simulink model "Simulink_one_rotor"  (R2024b)
settings: Solver=VariableStepAuto  StartTime=0.0  StopTime=0.5  RelTol=1e-3
settings Model: Creator=yuany  LastModifiedBy=yuany

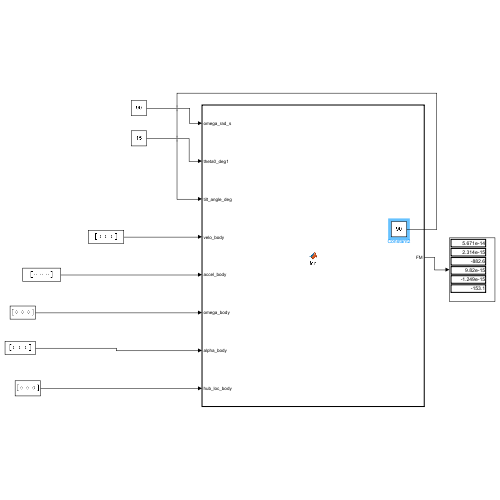
[thumbnail: Simulink's stored preview of the top-level diagram]
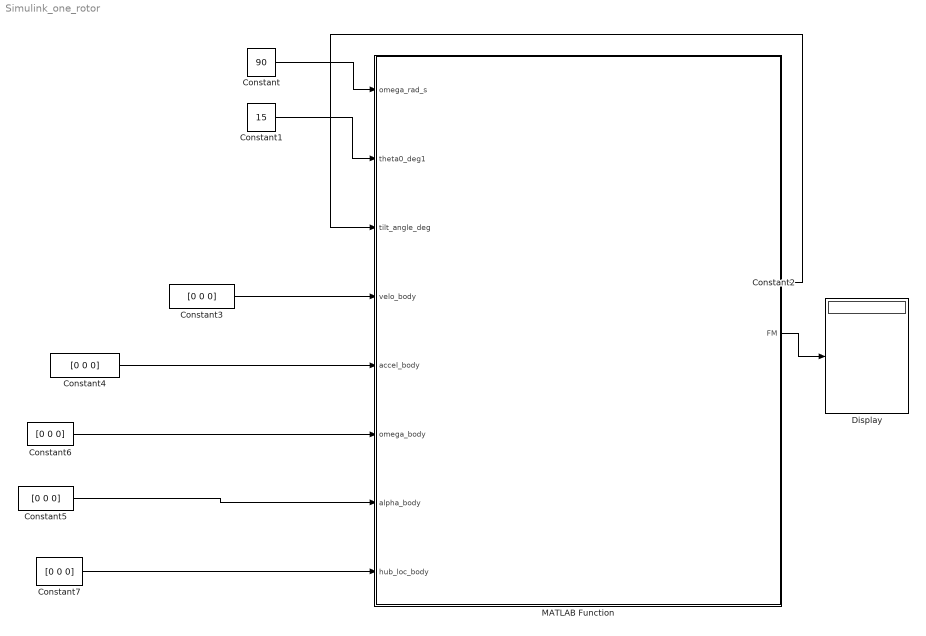
== system Simulink_one_rotor ==
  Constant : Constant  Value=90
  Constant1 : Constant  Value=15
  Constant2 : Constant  Value=90
  Constant{3..7} (5 alike) : Constant  Value=[0 0 0]
  Display : Display
  MATLAB Function : MATLAB Function  TreatAsAtomicUnit=on
  wires:
  Constant/1 -> MATLAB Function/1(omega_rad_s)
  Constant1/1 -> MATLAB Function/2(theta0_deg1)
  Constant2/1 -> MATLAB Function/3(tilt_angle_deg)
  Constant3/1 -> MATLAB Function/4(velo_body)
  Constant4/1 -> MATLAB Function/5(accel_body)
  Constant5/1 -> MATLAB Function/7(alpha_body)
  Constant6/1 -> MATLAB Function/6(omega_body)
  MATLAB Function/1(FM) -> Display/1
  Constant7/1 -> MATLAB Function/8(hub_loc_body)

== matlab function Simulink_one_rotor/MATLAB Function ==
  data: omega_rad_s input; FM output; theta0_deg1 input; tilt_angle_deg input; velo_body input; accel_body input; omega_body input; alpha_body input; hub_loc_body input
function FM = fcn(omega_rad_s, theta0_deg1, tilt_angle_deg, ... 
    velo_body, accel_body, omega_body, alpha_body, hub_loc_body) 
ff=load('rotor.mat');
rotor=ff.rotor;
velo_body = velo_body';
angular_velocity_body = omega_body';
acceleration_body = accel_body';
angular_acceleration_body = alpha_body';
rotor.omega=omega_rad_s;
rotor.tilt_angle_deg=tilt_angle_deg;
rotor.hub_loc=hub_loc_body';

%% Rotor definition
max_id = 6;

%% Control input
theta0_deg = theta0_deg1;

%% Solver options
max_iter = 40;
tol = 1e-10;
fd_step = 1e-4;
damping = 1.0;
min_damping = 0.15;
initial_guess = [zeros(2*rotor.Nb,1); 1.0];

%% Solve
[forces, converged, iter, residual, residual_norm, power, vi, ...
    beta0, dbeta0, beta_hist, dbeta_hist, alpha_hist] = ...
    rotor_bemt_trim_flat_codegen_ready( ...
        rotor, ...
        velo_body, angular_velocity_body, acceleration_body, angular_acceleration_body, ...
        theta0_deg, ...
        max_iter, tol, fd_step, damping, min_damping, initial_guess);

FM=forces;
end

function [forces, converged, iter, residual, residual_norm, power, vi, beta0, dbeta0, beta_hist, dbeta_hist, alpha_hist] = ...
    rotor_bemt_trim_flat_codegen_ready( ...
        rotor, ...
        velo_body, angular_velocity_body, acceleration_body, angular_acceleration_body, ...
        theta0_deg, ...
        max_iter, tol, fd_step, damping, min_damping, initial_guess)
% rotor_bemt_trim_flat_codegen_ready
%
% Code-generation-friendly BEMT + flap trim core.
%
% Runtime restrictions intentionally enforced:
%   - only one struct is used: rotor
%   - no state/options/info/aux/flow_state structs
%   - no try/catch
%   - no function_handle
%   - no griddedInterpolant
%   - no runtime file I/O
%   - no runtime text parsing / MAT loading
%
% Model selection is numeric:
%   rotor.airfoil_mode_code  : 1 linear, 2 lookup table
%   rotor.chord_mode_code    : 1 linear, 2 lookup table
%   rotor.chord_unit_code    : 1 meter, 2 c_over_R
%   rotor.pretwist_mode_code : 1 linear, 2 lookup table
%
% For lookup mode, the corresponding numeric arrays must already be stored
% in rotor before calling this function.

    x = initial_guess(:);
    converged = false;

    for iter = 1:max_iter
        [residual, forces, power, beta_hist, dbeta_hist, alpha_hist, ...
            Tb_average, V_inf, V_infy, V_z] = ...
            rotor_trim_residual_flat_codegen( ...
                x, rotor, ...
                velo_body, angular_velocity_body, acceleration_body, angular_acceleration_body, ...
                theta0_deg);

        resnorm = norm(residual);

        if resnorm < tol
            converged = true;
            break;
        end

        n = numel(x);
        J = zeros(n, n);
        for i = 1:n
            dx = fd_step * max(1.0, abs(x(i)));
            xp = x;
            xp(i) = xp(i) + dx;

            rp = rotor_trim_residual_flat_codegen( ...
                xp, rotor, ...
                velo_body, angular_velocity_body, acceleration_body, angular_acceleration_body, ...
                theta0_deg);

            J(:, i) = (rp - residual) / dx;
        end

        step = -J \ residual;

        alpha = damping;
        accepted = false;
        for ls = 1:8
            x_try = x + alpha * step;

            r_try = rotor_trim_residual_flat_codegen( ...
                x_try, rotor, ...
                velo_body, angular_velocity_body, acceleration_body, angular_acceleration_body, ...
                theta0_deg);

            if norm(r_try) < resnorm
                x = x_try;
                accepted = true;
                break;
            end

            alpha = alpha * 0.5;
        end

        if ~accepted
            x = x + min_damping * step;
        end
    end

    [residual, forces, power, beta_hist, dbeta_hist, alpha_hist, ...
        Tb_average, V_inf, V_infy, V_z] = ...
        rotor_trim_residual_flat_codegen( ...
            x, rotor, ...
            velo_body, angular_velocity_body, acceleration_body, angular_acceleration_body, ...
            theta0_deg);

    residual_norm = norm(residual);
    beta0 = x(1:rotor.Nb);
    dbeta0 = x(rotor.Nb+1:2*rotor.Nb);
    vi = x(end);

    %#ok<NASGU>
    %#ok<ASGLU>
end


function [residual, forces, power, beta_hist, dbeta_hist, alpha_hist, ...
          Tb_average, V_inf, V_infy, V_z] = ...
    rotor_trim_residual_flat_codegen( ...
        x, rotor, ...
        velo_body, angular_velocity_body, acceleration_body, angular_acceleration_body, ...
        theta0_deg)

    Nb = rotor.Nb;

    beta0 = x(1:Nb);
    dbeta0 = x(Nb+1:2*Nb);
    vi = x(end);

    [forces, beta_hist, dbeta_hist, power, alpha_hist, ...
        Tb_average, V_inf, V_infy, V_z] = ...
        rotor_forces_one_rev_flat_codegen( ...
            beta0, dbeta0, vi, rotor, ...
            velo_body, angular_velocity_body, acceleration_body, angular_acceleration_body, ...
            theta0_deg);

    residual = zeros(2*Nb + 1, 1);
    residual(1:Nb) = beta_hist(end, :).'-beta0(:);
    residual(Nb+1:2*Nb) = dbeta_hist(end, :).'-dbeta0(:);

    residual(end) = ( ...
        Tb_average + ...
        2*rotor.rho*pi*rotor.R^2 * ...
        sqrt((V_z + vi)^2 + V_inf^2 + V_infy^2) * vi ...
        ) / (rotor.rho*pi*rotor.R^2*rotor.omega^2);
end


function [forces, beta_hist, dbeta_hist, power, alpha_hist, ...
          Tb_average, V_inf, V_infy, V_z] = ...
    rotor_forces_one_rev_flat_codegen( ...
        beta0, dbeta0, vi, rotor, ...
        velo_body, angular_velocity_body, acceleration_body, angular_acceleration_body, ...
        theta0_deg)

    rho = rotor.rho;
    R = rotor.R;
    Nb = rotor.Nb;
    omega = rotor.omega * rotor.rotational_direction;
    I_beta = rotor.I_beta;
    k_beta = rotor.k_beta;

    n_be = rotor.n_be;
    n_az = rotor.n_az;
    root_cutout = rotor.root_cutout;

    dpsi = 2*pi / n_az;
    dt = dpsi / abs(omega);
    dr_phys = (R - root_cutout*R) / n_be;

    alpha_hist = zeros(n_az, n_be);

    veloo = velo_body(:) + cross(angular_velocity_body(:), rotor.hub_loc(:));

    tilt = deg2rad(rotor.tilt_angle_deg);
    T_body2disc = [ sin(tilt)  0  cos(tilt); ...
                    0          1  0; ...
                   -cos(tilt)  0  sin(tilt) ];
    T_disc2body = T_body2disc';

    v_disc = T_body2disc * veloo;
    w_disc = T_body2disc * angular_velocity_body(:);
    a_disc = T_body2disc * acceleration_body(:);
    ang_acc_disc = T_body2disc * angular_acceleration_body(:);

    ppp = w_disc(1);
    qqq = w_disc(2);
    uuu = v_disc(1);
    vvv = v_disc(2);
    aaw = a_disc(3);
    aap = ang_acc_disc(1);
    aaq = ang_acc_disc(2);

    theta0 = deg2rad(theta0_deg);

    V_inf  = v_disc(1);
    V_infy = v_disc(2);
    V_z    = v_disc(3);
    velocity1 = [V_inf; V_infy; V_z];

    beta_hist = zeros(n_az+1, Nb);
    dbeta_hist = zeros(n_az+1, Nb);
    beta_hist(1, :) = beta0(:).';
    dbeta_hist(1, :) = dbeta0(:).';

    Tb_average = 0;
    Hb_average = 0;
    Sb_average = 0;
    Torque_average = 0;
    M_average = 0;
    L_average = 0;

    for blade = 1:Nb
        beta_dot = dbeta_hist(1, blade);

        for iaz = 1:n_az
            Tb_new = 0;
            Hb_new = 0;
            Sb_new = 0;
            M_A = 0;
            M_torque = 0;

            Az = rotor.rotational_direction * ((iaz-1)*dpsi + (blade-1)*2*pi/Nb);

            T_az = [-cos(Az) -sin(Az)  0; ...
                     sin(Az) -cos(Az)  0; ...
                     0        0        1];
            T_az_inv = T_az';

            beta_now = beta_hist(iaz, blade);
            T_flap = [ cos(beta_now) 0 -sin(beta_now); ...
                       0             1  0; ...
                       sin(beta_now) 0  cos(beta_now) ];
            T_flap_inv = T_flap';

            velocity2 = T_az * velocity1;
            w_shaft = T_az * w_disc + [0; 0; omega];
            w_blade = T_flap * w_shaft + [0; beta_dot; 0];
            velocity_blade_root = T_flap * velocity2;

            for iz = 1:n_be
                x = root_cutout + (1-root_cutout)/(2*n_be) + (iz-1)*(1-root_cutout)/n_be;
                r = x * R;

                v_blade_elem = velocity_blade_root + cross(w_blade, [r; 0; 0]);
                pretwist_deg = eval_pretwist_flat_codegen(rotor, x);
                theta = theta0 + deg2rad(pretwist_deg);

                V_n = v_blade_elem(3) - vi*cos(beta_now);
                vt  = rotor.rotational_direction * v_blade_elem(2);

                phi_new = atan2(V_n, vt);
                alpha_new = theta + phi_new;

                if blade == 1
                    alpha_hist(iaz, iz) = alpha_new;
                end

                Mach = sqrt(V_n^2 + vt^2) / 340;
                [CL, CD] = eval_airfoil_flat_codegen(rotor, x, rad2deg(alpha_new), Mach);
                chord_val = eval_chord_flat_codegen(rotor, x);

                qdyn = 0.5 * rho * (vt^2 + (vi - V_n)^2);
                dL = qdyn * chord_val * dr_phys * CL;
                dD = qdyn * chord_val * dr_phys * CD;

                T_be = -(dL*cos(phi_new) + dD*sin(phi_new));
                D_be = -rotor.rotational_direction*dD*cos(phi_new) + ...
                        rotor.rotational_direction*dL*sin(phi_new);

                M_torque = M_torque + D_be*r;

                blade_force = [0; D_be; T_be];
                blade_force = T_flap_inv * blade_force;
                blade_force = T_az_inv * blade_force;

                Tb_new = Tb_new + blade_force(3);
                Hb_new = Hb_new + blade_force(1);
                Sb_new = Sb_new + blade_force(2);
                M_A = M_A + blade_force(3)*r;
            end

            Tb_average = Tb_average + Tb_new / n_az;
            Hb_average = Hb_average + Hb_new / n_az;
            Sb_average = Sb_average + Sb_new / n_az;
            Torque_average = Torque_average + M_torque / n_az;

            M_CF = -omega^2 * I_beta * beta_now;
            M_R  = -k_beta * beta_now;
            M_cor = -2 * I_beta * (ppp*omega*cos(Az) - qqq*omega*sin(Az));
            M_ba = I_beta * (aap*sin(Az) + aaq*cos(Az));
            M_bl = 1.5 * (aaw - uuu*qqq + ppp*vvv);

            M_average = M_average + M_R*cos(Az)/n_az;
            L_average = L_average + M_R*sin(Az)/n_az;

            beta_2dot = (M_A + M_CF + M_R + M_cor + M_ba + M_bl) / I_beta;
            beta_dot = beta_dot + beta_2dot * dt;

            dbeta_hist(iaz+1, blade) = beta_dot;
            beta_hist(iaz+1, blade) = beta_hist(iaz, blade) + beta_dot * dt;
        end
    end

    forces_disc = [Hb_average; Sb_average; Tb_average];
    forces_body = T_disc2body * forces_disc;

    moments_disc = [L_average; M_average; Torque_average];
    moments_body_from_disc = T_disc2body * moments_disc;

    aero_moment_from_hub = cross(rotor.hub_loc(:), forces_body(:));

    forces = zeros(6,1);
    forces(1:3) = forces_body;
    forces(4:6) = moments_body_from_disc + aero_moment_from_hub;

    power = abs(Torque_average) * abs(omega);
end


function [CL, CD] = eval_airfoil_flat_codegen(rotor, x, alpha_deg, Mach)
    idx = pick_section_index_flat_codegen(rotor.section_r_end, x);
    airfoil_id = rotor.section_airfoil_id(idx);

    if rotor.airfoil_mode_code == 1
        alpha_eff_rad = deg2rad(alpha_deg - rotor.airfoil_alpha0_deg(airfoil_id));
        CL = rotor.airfoil_a0(airfoil_id) * alpha_eff_rad;
        CD = rotor.airfoil_cd0(airfoil_id) + rotor.airfoil_k(airfoil_id) * CL^2;
    else
        CL = interp2_bilinear_clamped_flat_codegen( ...
            rotor.airfoil_alpha_grid, rotor.airfoil_mach_grid, ...
            rotor.airfoil_cl_table(:,:,airfoil_id), alpha_deg, Mach);

        CD = interp2_bilinear_clamped_flat_codegen( ...
            rotor.airfoil_alpha_grid, rotor.airfoil_mach_grid, ...
            rotor.airfoil_cd_table(:,:,airfoil_id), alpha_deg, Mach);
    end
end


function chord_m = eval_chord_flat_codegen(rotor, x)
    if rotor.chord_mode_code == 1
        s = (x - rotor.root_cutout) / (1 - rotor.root_cutout);
        s = min(max(s, 0), 1);
        raw = rotor.chord_root_value + s * (rotor.chord_tip_value - rotor.chord_root_value);
    else
        raw = interp1_linear_clamped_flat_codegen(rotor.chord_x_grid, rotor.chord_lookup_val, x);
    end

    if rotor.chord_unit_code == 1
        chord_m = raw;
    else
        chord_m = raw * rotor.R;
    end
end


function pretwist_deg = eval_pretwist_flat_codegen(rotor, x)
    if rotor.pretwist_mode_code == 1
        s = (x - rotor.root_cutout) / (1 - rotor.root_cutout);
        s = min(max(s, 0), 1);
        pretwist_deg = rotor.pretwist_root_deg + ...
            s * (rotor.pretwist_tip_deg - rotor.pretwist_root_deg);
    else
        pretwist_deg = interp1_linear_clamped_flat_codegen( ...
            rotor.pretwist_x_grid, rotor.pretwist_lookup_val, x);
    end
end


function idx = pick_section_index_flat_codegen(section_r_end, x)
    idx = numel(section_r_end);
    for k = 1:numel(section_r_end)
        if x <= section_r_end(k)
            idx = k;
            break;
        end
    end
end


function y = interp1_linear_clamped_flat_codegen(xg, yg, xq)
    n = numel(xg);

    if xq <= xg(1)
        y = yg(1);
        return;
    end
    if xq >= xg(n)
        y = yg(n);
        return;
    end

    i = 1;
    for k = 1:n-1
        if xq >= xg(k) && xq <= xg(k+1)
            i = k;
            break;
        end
    end

    t = (xq - xg(i)) / (xg(i+1) - xg(i));
    y = (1-t)*yg(i) + t*yg(i+1);
end


function zq = interp2_bilinear_clamped_flat_codegen(xg, yg, Z, xq, yq)
    nx = numel(xg);
    ny = numel(yg);

    if xq <= xg(1)
        ix = 1;
        tx = 0;
    elseif xq >= xg(nx)
        ix = nx - 1;
        tx = 1;
    else
        ix = 1;
        for k = 1:nx-1
            if xq >= xg(k) && xq <= xg(k+1)
                ix = k;
                break;
            end
        end
        tx = (xq - xg(ix)) / (xg(ix+1) - xg(ix));
    end

    if yq <= yg(1)
        iy = 1;
        ty = 0;
    elseif yq >= yg(ny)
        iy = ny - 1;
        ty = 1;
    else
        iy = 1;
        for k = 1:ny-1
            if yq >= yg(k) && yq <= yg(k+1)
                iy = k;
                break;
            end
        end
        ty = (yq - yg(iy)) / (yg(iy+1) - yg(iy));
    end

    z11 = Z(ix,   iy);
    z21 = Z(ix+1, iy);
    z12 = Z(ix,   iy+1);
    z22 = Z(ix+1, iy+1);

    zq = (1-tx)*(1-ty)*z11 + tx*(1-ty)*z21 + (1-tx)*ty*z12 + tx*ty*z22;
end
